simulink model "mco12082024simulink"  (R2012b)
settings: Solver=ode45  StartTime=0.0  StopTime=120  RelTol=1e-3
values from neighbouring files (symbols this model uses):
  ki = kp/ti    [exemplo3.m]    (also in omc140824.m = kp/Ti)
  kp = (2*tau+theta)/(2*k*lambda)    [exemplo3.m]    (also in omc140824.m)
libraries: cstblocks x1
settings Model: Creator=rreis  LastModifiedBy=Henrique.Alles

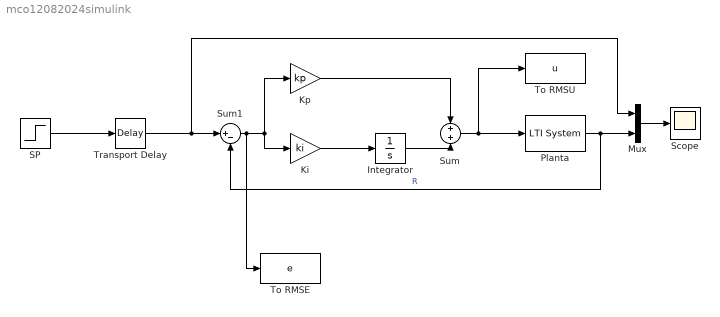
== system mco12082024simulink ==
  Integrator : Integrator
  Ki : Gain  Gain=ki
  Kp : Gain  Gain=kp
  Mux : Mux  Inputs=2
  Planta : cstblocks/LTI System  sys=G  IC=[]
  SP : Step  Time=0  SampleTime=0.1
  Scope : Scope
      settings: ShowLegends=on
  Sum : Sum
  Sum1 : Sum  Inputs=|+-
  To RMSE : ToWorkspace  VariableName=e  SampleTime=-1
  To RMSU : ToWorkspace  VariableName=u  SampleTime=-1
  Transport Delay : TransportDelay  DelayTime=2
  wires:
  Integrator/1 -> Sum/2
  Sum/1 -> To RMSU/1, Planta/1
  Ki/1 -> Integrator/1
  Kp/1 -> Sum/1
  Sum1/1 -> To RMSE/1, Kp/1, Ki/1
  Planta/1 -> Sum1/2, Mux/2  "R"
  Mux/1 -> Scope/1
  Transport Delay/1 -> Mux/1, Sum1/1
  SP/1 -> Transport Delay/1
